simulink model "Second_Order_System_Adjustment_With_First_Order_Controller"  (R2013b)
settings: Solver=ode45  StartTime=0.0  StopTime=50  RelTol=1e-3
values from neighbouring files (symbols this model uses):
  A = [1 1 6]    [SecondOrderSystemAdjustmentWithFirstOrderController.m]
  Am = [1 9 26 24]    [SecondOrderSystemAdjustmentWithFirstOrderController.m]
  B = [1 2]    [SecondOrderSystemAdjustmentWithFirstOrderController.m]
  Bm = [1 24]    [SecondOrderSystemAdjustmentWithFirstOrderController.m]
  Gamma1 = [k]/2    [SecondOrderSystemAdjustmentWithFirstOrderController.m]
  Gamma2 = [k]/4    [SecondOrderSystemAdjustmentWithFirstOrderController.m]
  Gamma3 = [-k]    [SecondOrderSystemAdjustmentWithFirstOrderController.m]
settings Model: Creator=MMSA  LastModifiedBy=MMSA
settings SolverCC: ZeroCrossAlgorithm=Adaptive  PositivePriorityOrder=on
settings DataIOCC: LimitDataPoints=off
settings HardwareCC: ProdBitPerPointer=64  ProdHWDeviceType=Generic->64-bit Embedded Processor (LLP64)

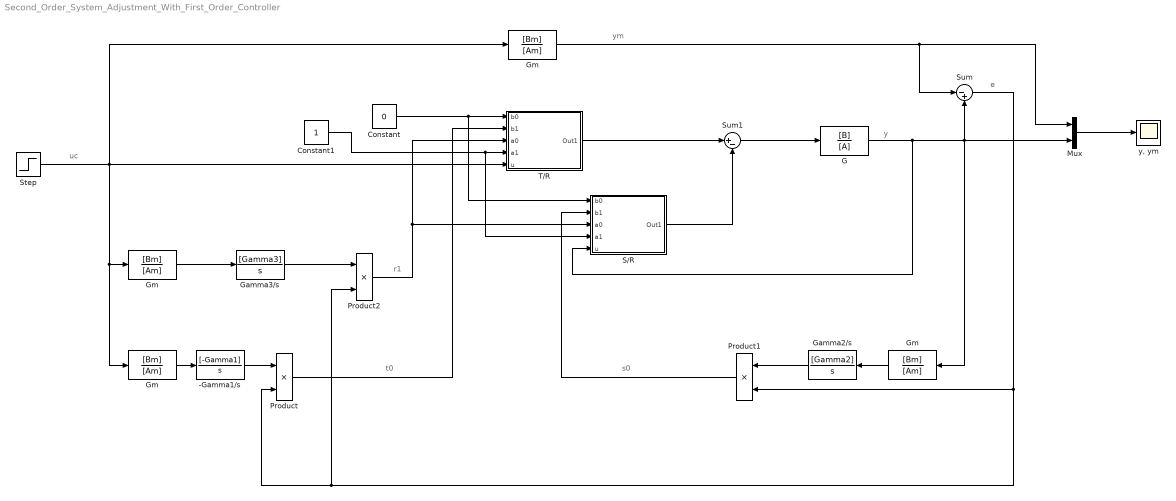
== system Second_Order_System_Adjustment_With_First_Order_Controller ==
  note: uc
  note: r1
  note: t0
  note: s0
  note: e
  note: y
  note: ym
  " Gm " : TransferFcn  Numerator=[Bm]  Denominator=[Am]
  -Gamma1/s : TransferFcn  Numerator=[-Gamma1]  Denominator=[1 0]
  Constant : Constant  Value=0
  Constant1 : Constant
  G : TransferFcn  Numerator=[B]  Denominator=[A]
  Gamma2/s : TransferFcn  Numerator=[Gamma2]  Denominator=[1 0]
  Gamma3/s : TransferFcn  Numerator=[Gamma3]  Denominator=[1 0]
  Gm : TransferFcn  Numerator=[Bm]  Denominator=[Am]
  "Gm " : TransferFcn  Numerator=[Bm]  Denominator=[Am]
  "Gm " : TransferFcn  Numerator=[Bm]  Denominator=[Am]
  Mux : Mux  Inputs=2
  Product : Product
  Product1 : Product
  Product2 : Product
  S/R : Subsystem
  Step : Step  Time=0  SampleTime=0
  Sum : Sum  Inputs=|-+
  Sum1 : Sum  Inputs=|+-
  T/R : Subsystem
  "y, ym" : Scope
      settings: TickLabels=on  ShowLegends=on  YMin=1.75  Decimation=10  SampleInput=on
  wires:
  Step/1 -> "Gm "/1, "Gm "/1, Gm/1, T/R/5(u)
  Mux/1 -> "y, ym"/1
  Gm/1 -> Sum/1, Mux/1
  G/1 -> S/R/5(u), " Gm "/1, Sum/2, Mux/2
  "Gm "/1 -> -Gamma1/s/1
  -Gamma1/s/1 -> Product/1
  " Gm "/1 -> Gamma2/s/1
  Gamma2/s/1 -> Product1/1
  "Gm "/1 -> Gamma3/s/1
  Gamma3/s/1 -> Product2/1
  Sum1/1 -> G/1
  T/R/1(Out1) -> Sum1/1
  Constant/1 -> S/R/1(b0), T/R/1(b0)
  Product/1 -> T/R/2(b1)
  Constant1/1 -> S/R/4(a1), T/R/4(a1)
  Product2/1 -> S/R/3(a0), T/R/3(a0)
  S/R/1(Out1) -> Sum1/2
  Product1/1 -> S/R/2(b1)
  Sum/1 -> Product1/2, Product2/2, Product/2

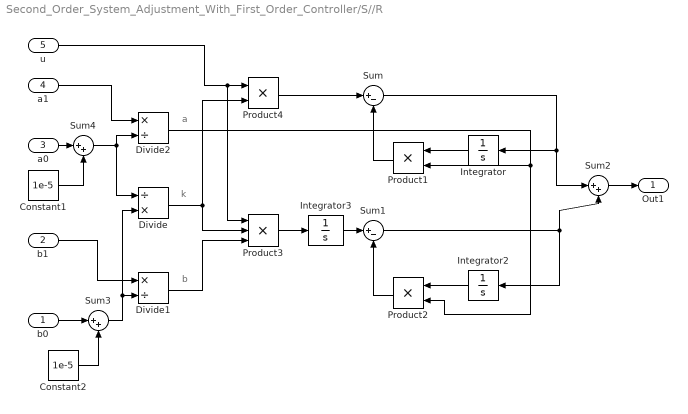
== system Second_Order_System_Adjustment_With_First_Order_Controller/S//R ==
  note: b
  note: a
  note: k
  b0 : Inport
  b1 : Inport  Port=2
  a0 : Inport  Port=3
  a1 : Inport  Port=4
  u : Inport  Port=5
  Constant1 : Constant  Value=1e-5
  Constant2 : Constant  Value=1e-5
  Divide : Product  Inputs=/*
  Divide1 : Product  Inputs=*/
  Divide2 : Product  Inputs=*/
  Integrator : Integrator
  Integrator2 : Integrator
  Integrator3 : Integrator
  Product1 : Product
  Product2 : Product
  Product3 : Product  Inputs=3
  Product4 : Product
  Sum : Sum  Inputs=|+-
  Sum1 : Sum  Inputs=|+-
  Sum2 : Sum  Inputs=|++
  Sum3 : Sum  Inputs=|++
  Sum4 : Sum  Inputs=|++
  Out1 : Outport
  wires:
  Integrator/1 -> Product1/1
  Product1/1 -> Sum/2
  Sum/1 -> Sum2/1, Integrator/1
  Product4/1 -> Sum/1
  b1/1 -> Divide1/1
  a1/1 -> Divide2/1
  Divide2/1 -> Product2/2, Product1/2
  Divide1/1 -> Product3/3
  Integrator2/1 -> Product2/1
  Product2/1 -> Sum1/2
  Sum1/1 -> Sum2/2, Integrator2/1
  Integrator3/1 -> Sum1/1
  Product3/1 -> Integrator3/1
  Divide/1 -> Product4/2, Product3/2
  u/1 -> Product4/1, Product3/1
  Sum2/1 -> Out1/1
  Constant2/1 -> Sum3/2
  b0/1 -> Sum3/1
  Sum3/1 -> Divide/2, Divide1/2
  a0/1 -> Sum4/1
  Sum4/1 -> Divide2/2, Divide/1
  Constant1/1 -> Sum4/2

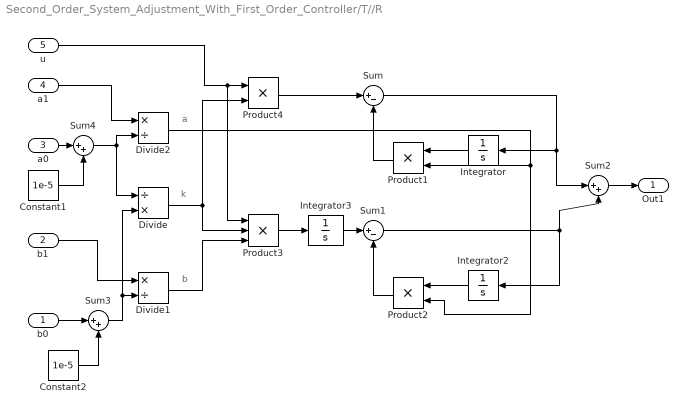
== system Second_Order_System_Adjustment_With_First_Order_Controller/T//R ==
  note: b
  note: a
  note: k
  b0 : Inport
  b1 : Inport  Port=2
  a0 : Inport  Port=3
  a1 : Inport  Port=4
  u : Inport  Port=5
  Constant1 : Constant  Value=1e-5
  Constant2 : Constant  Value=1e-5
  Divide : Product  Inputs=/*
  Divide1 : Product  Inputs=*/
  Divide2 : Product  Inputs=*/
  Integrator : Integrator
  Integrator2 : Integrator
  Integrator3 : Integrator
  Product1 : Product
  Product2 : Product
  Product3 : Product  Inputs=3
  Product4 : Product
  Sum : Sum  Inputs=|+-
  Sum1 : Sum  Inputs=|+-
  Sum2 : Sum  Inputs=|++
  Sum3 : Sum  Inputs=|++
  Sum4 : Sum  Inputs=|++
  Out1 : Outport
  wires:
  Integrator/1 -> Product1/1
  Product1/1 -> Sum/2
  Sum/1 -> Sum2/1, Integrator/1
  Product4/1 -> Sum/1
  b1/1 -> Divide1/1
  a1/1 -> Divide2/1
  Divide2/1 -> Product2/2, Product1/2
  Divide1/1 -> Product3/3
  Integrator2/1 -> Product2/1
  Product2/1 -> Sum1/2
  Sum1/1 -> Sum2/2, Integrator2/1
  Integrator3/1 -> Sum1/1
  Product3/1 -> Integrator3/1
  Divide/1 -> Product4/2, Product3/2
  u/1 -> Product4/1, Product3/1
  Sum2/1 -> Out1/1
  Constant2/1 -> Sum3/2
  b0/1 -> Sum3/1
  Sum3/1 -> Divide/2, Divide1/2
  a0/1 -> Sum4/1
  Sum4/1 -> Divide2/2, Divide/1
  Constant1/1 -> Sum4/2
